simulink model "soc_swhw_fpga"  (R2021a)
settings: Solver=VariableStepAuto  StartTime=0.0  StopTime=stopTime  RelTol=1e-3  EnableMultiTasking=on
PreLoadFcn:
  | hsb.blkcb2.defineTypes;
undefined symbols (not defined in the file): a, b, Bias1, Bias2, c, frameSize, jsin, LUT_Z0, LUT_Z1, NumBits1, NumBits2, quantizationBits, sampleTime, SF, Slope1, Slope2
libraries: simulink x42, hdlsllib x24, embreciprocals x4, hwlogicconnlib x4, dsphdlxfrm x2, dsphdlmathfun x1
(part 2 of 2)

== system soc_swhw_fpga/FPGA Algorithm Wrapper/Output Adapter/Zero Chop ==
  validIn : Inport
  dataIn : Inport  Port=2
  AND : Logic  AllPortsSameDT=off  OutDataTypeStr=boolean
  Compare To Constant : simulink/Logic and Bit Operations/Compare To Constant  relop=<=  const=frameSize  OutDataTypeStr=boolean
  Compare To Constant1 : simulink/Logic and Bit Operations/Compare To Constant  relop=~=  const=0  OutDataTypeStr=boolean
  Enabled Counter1 : Subsystem  TreatAsAtomicUnit=on  mask(Counter){maxCount=(2 ^ (floor(log2(frameSize)) + 1)), sampleTime=-1}
      mask prompts: maxCount "Maximum count:"; sampleTime "Sample Time:"
  validOut : Outport
  dataOut : Outport  Port=2
  wires:
  AND/1 -> validOut/1
  Compare To Constant1/1 -> AND/2
  Enabled Counter1/1(count) -> Compare To Constant/1, Compare To Constant1/1
  Compare To Constant/1 -> AND/1
  validIn/1 -> Enabled Counter1/1(en)
  dataIn/1 -> dataOut/1

== system soc_swhw_fpga/FPGA Algorithm Wrapper/Feature Extraction/VAD/Enabled Counter ==
  en : Inport
  Compare To Constant : simulink/Logic and Bit Operations/Compare To Constant  relop===  const=maxCount  OutDataTypeStr=boolean
  Constant1 : Constant  Value=0  OutDataTypeStr=uint(floor(log2(maxCount))+1)  SampleTime=-1
  Delay One Step : Delay  DelayLength=1  InitialCondition=0
  Delay One Step1 : Delay  DelayLength=1  InitialCondition=0
  Increment Real World : simulink/Additional Math & Discrete/Additional Math: Increment - Decrement/Increment Real World
      settings: SourceProductBaseCode=SL
  Multiport Switch : MultiPortSwitch  DataPortOrder=Zero-based contiguous  Inputs=2  zeroidx=on
  Multiport Switch1 : MultiPortSwitch  DataPortOrder=Zero-based contiguous  Inputs=2  zeroidx=on
  Multiport Switch2 : MultiPortSwitch  DataPortOrder=Zero-based contiguous  Inputs=2  zeroidx=on
  count : Outport
  wires:
  en/1 -> Multiport Switch1/1, Multiport Switch/1
  Increment Real World/1 -> Multiport Switch/3
  Multiport Switch/1 -> Multiport Switch2/2, Multiport Switch1/3, Compare To Constant/1
  Delay One Step/1 -> Multiport Switch/2, Increment Real World/1
  Compare To Constant/1 -> Multiport Switch2/1
  Delay One Step1/1 -> Multiport Switch1/2
  Multiport Switch1/1 -> count/1, Delay One Step1/1
  Multiport Switch2/1 -> Delay One Step/1
  Constant1/1 -> Multiport Switch2/3

== system soc_swhw_fpga/FPGA Algorithm Wrapper/Feature Extraction/VAD/Pos Edge Detector ==
  q : Inport
  AND : Logic  AllPortsSameDT=off  OutDataTypeStr=boolean
  Delay1 : Delay  DelayLength=1
  XOR : Logic  Operator=XOR  AllPortsSameDT=off  OutDataTypeStr=boolean
  detected : Outport
  wires:
  XOR/1 -> AND/1
  Delay1/1 -> XOR/2
  q/1 -> XOR/1, AND/2, Delay1/1
  AND/1 -> detected/1

== system soc_swhw_fpga/FPGA Algorithm Wrapper/Feature Extraction/VAD/Pos Edge Detector1 ==
  q : Inport
  AND : Logic  AllPortsSameDT=off  OutDataTypeStr=boolean
  Delay1 : Delay  DelayLength=1
  XOR : Logic  Operator=XOR  AllPortsSameDT=off  OutDataTypeStr=boolean
  detected : Outport
  wires:
  XOR/1 -> AND/1
  Delay1/1 -> XOR/2
  q/1 -> XOR/1, AND/2, Delay1/1
  AND/1 -> detected/1

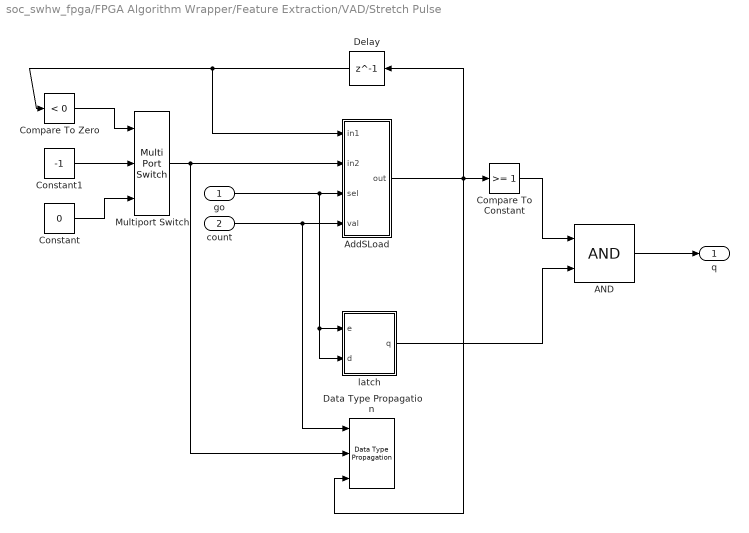
== system soc_swhw_fpga/FPGA Algorithm Wrapper/Feature Extraction/VAD/Stretch Pulse ==
  go : Inport  OutDataTypeStr=boolean
  count : Inport  Port=2
  AND : Logic  AllPortsSameDT=off  OutDataTypeStr=boolean
  AddSLoad : Subsystem
  Compare To Constant : simulink/Logic and Bit Operations/Compare To Constant  relop=>=  const=1  OutDataTypeStr=boolean
  Compare To Zero : simulink/Logic and Bit Operations/Compare To Zero  relop=<  OutDataTypeStr=boolean
  Constant : Constant  Value=0  OutDataTypeStr=fixdt(0,1,0)  SampleTime=-1
  Constant1 : Constant  Value=-1  OutDataTypeStr=fixdt(1,2,0)  SampleTime=-1
  Data Type Propagation : simulink/Signal Attributes/Data Type Propagation  PropDataType=fixdt(1, 16)  IfRefDouble=double  IfRefSingle=single  IsSigned=IsSigned1 or IsSigned2  NumBitsBase=max([NumBits1 NumBits2])  NumBitsMult=1  NumBitsAdd=1  NumBitsAllowFinal=1:128  PropScaling=2^-10  ValuesUsedBestPrec=[5 -7]  SlopeBase=max([Slope1 Slope2])  SlopeMult=1  SlopeAdd=0  BiasBase=Bias1+Bias2  BiasMult=1  BiasAdd=0
      settings: SourceProductBaseCode=SL
  Delay : Delay  DelayLength=1
  Multiport Switch : MultiPortSwitch  DataPortOrder=Zero-based contiguous  Inputs=2  zeroidx=on
  latch : Subsystem
  q : Outport
  wires:
  AddSLoad/1(out) -> Data Type Propagation/3, Compare To Constant/1, Delay/1
  Constant/1 -> Multiport Switch/3
  Delay/1 -> Compare To Zero/1, AddSLoad/1(in1)
  latch/1(q) -> AND/2
  Constant1/1 -> Multiport Switch/2
  Multiport Switch/1 -> Data Type Propagation/2, AddSLoad/2(in2)
  Compare To Zero/1 -> Multiport Switch/1
  Compare To Constant/1 -> AND/1
  go/1 -> latch/1(e), latch/2(d), AddSLoad/3(sel)
  AND/1 -> q/1
  count/1 -> Data Type Propagation/1, AddSLoad/4(val)

== system soc_swhw_fpga/FPGA Algorithm Wrapper/Feature Extraction/VAD/bitFuse ==
  q : Inport
  Delay : Delay  DelayLength=1
  Multiport Switch : MultiPortSwitch  DataPortOrder=Zero-based contiguous  Inputs=2  zeroidx=on
  tripped : Outport
  wires:
  Delay/1 -> Multiport Switch/3, Multiport Switch/1
  Multiport Switch/1 -> tripped/1, Delay/1
  q/1 -> Multiport Switch/2

== system soc_swhw_fpga/FPGA Algorithm Wrapper/Feature Extraction/aPosterioriSNR/Frame Fuse ==
  validIn : Inport
  1bit Counter : hdlsllib/Sources/HDL Counter  CountType=Count limited  CountInit=0  CountStep=1  CountMax=1  CountFromType=Initial value  CountFrom=0  CountResetPort=off  CountLoadPort=off  CountEnbPort=on  CountDirPort=off  CountHitOutputPort=off  CountDataType=Unsigned  CountWordLen=1  CountFracLen=0  CountSampTime=1
  Constant : Constant  Value=0  OutDataTypeStr=fixdt(0, 1, 0)  SampleTime=sampleTime
  Delay : Delay  DelayLength=1
  Multiport Switch : MultiPortSwitch  DataPortOrder=Zero-based contiguous  Inputs=2  zeroidx=on
  Pulse Divider : Subsystem  mask{N=ceil(log2(frameSize)) - 1}
  tripped : Outport
  wires:
  1bit Counter/1 -> Delay/1
  Constant/1 -> Multiport Switch/3
  Delay/1 -> Multiport Switch/1, tripped/1
  Pulse Divider/1(q) -> Multiport Switch/2
  validIn/1 -> Pulse Divider/1(In1)
  Multiport Switch/1 -> 1bit Counter/1

== system soc_swhw_fpga/FPGA Algorithm Wrapper/Feature Extraction/aPosterioriSNR/Zero Eliminator ==
  in : Inport
  Compare To Zero : simulink/Logic and Bit Operations/Compare To Zero  relop===  OutDataTypeStr=boolean
  Constant : Constant  OutDataTypeStr=fixdt(0, 1, 0)
  Multiport Switch6 : MultiPortSwitch  DataPortOrder=Zero-based contiguous  Inputs=2  zeroidx=on
  out : Outport
  wires:
  Multiport Switch6/1 -> out/1
  Compare To Zero/1 -> Multiport Switch6/1
  Constant/1 -> Multiport Switch6/3
  in/1 -> Multiport Switch6/2, Compare To Zero/1

== system soc_swhw_fpga/FPGA Algorithm Wrapper/Feature Extraction/aPosterioriSNR/Zero Eliminator1 ==
  in : Inport
  Compare To Zero : simulink/Logic and Bit Operations/Compare To Zero  relop===  OutDataTypeStr=boolean
  Constant : Constant  OutDataTypeStr=fixdt(0, 1, 0)
  Multiport Switch6 : MultiPortSwitch  DataPortOrder=Zero-based contiguous  Inputs=2  zeroidx=on
  out : Outport
  wires:
  in/1 -> Compare To Zero/1, Multiport Switch6/2
  Constant/1 -> Multiport Switch6/3
  Compare To Zero/1 -> Multiport Switch6/1
  Multiport Switch6/1 -> out/1

== system soc_swhw_fpga/FPGA Algorithm Wrapper/Feature Extraction/aPrioriSNR/Frame Fuse ==
  validIn : Inport
  1bit Counter : hdlsllib/Sources/HDL Counter  CountType=Count limited  CountInit=0  CountStep=1  CountMax=1  CountFromType=Initial value  CountFrom=0  CountResetPort=off  CountLoadPort=off  CountEnbPort=on  CountDirPort=off  CountHitOutputPort=off  CountDataType=Unsigned  CountWordLen=1  CountFracLen=0  CountSampTime=1
  Constant : Constant  Value=0  OutDataTypeStr=fixdt(0, 1, 0)  SampleTime=sampleTime
  Delay : Delay  DelayLength=1
  Multiport Switch : MultiPortSwitch  DataPortOrder=Zero-based contiguous  Inputs=2  zeroidx=on
  Pulse Divider : Subsystem  mask{N=ceil(log2(frameSize)) - 1}
  tripped : Outport
  wires:
  1bit Counter/1 -> Delay/1
  Constant/1 -> Multiport Switch/3
  Delay/1 -> Multiport Switch/1, tripped/1
  Pulse Divider/1(q) -> Multiport Switch/2
  validIn/1 -> Pulse Divider/1(In1)
  Multiport Switch/1 -> 1bit Counter/1

== system soc_swhw_fpga/FPGA Algorithm Wrapper/Input Adapter/Hamming Window/Enabled Counter ==
  en : Inport
  Compare To Constant : simulink/Logic and Bit Operations/Compare To Constant  relop===  const=maxCount  OutDataTypeStr=boolean
  Constant1 : Constant  Value=0  OutDataTypeStr=uint(floor(log2(maxCount))+1)  SampleTime=-1
  Delay One Step : Delay  DelayLength=1  InitialCondition=0
  Delay One Step1 : Delay  DelayLength=1  InitialCondition=0
  Increment Real World : simulink/Additional Math & Discrete/Additional Math: Increment - Decrement/Increment Real World
      settings: SourceProductBaseCode=SL
  Multiport Switch : MultiPortSwitch  DataPortOrder=Zero-based contiguous  Inputs=2  zeroidx=on
  Multiport Switch1 : MultiPortSwitch  DataPortOrder=Zero-based contiguous  Inputs=2  zeroidx=on
  Multiport Switch2 : MultiPortSwitch  DataPortOrder=Zero-based contiguous  Inputs=2  zeroidx=on
  count : Outport
  wires:
  en/1 -> Multiport Switch1/1, Multiport Switch/1
  Increment Real World/1 -> Multiport Switch/3
  Multiport Switch/1 -> Multiport Switch2/2, Multiport Switch1/3, Compare To Constant/1
  Delay One Step/1 -> Increment Real World/1, Multiport Switch/2
  Compare To Constant/1 -> Multiport Switch2/1
  Delay One Step1/1 -> Multiport Switch1/2
  Multiport Switch1/1 -> count/1, Delay One Step1/1
  Multiport Switch2/1 -> Delay One Step/1
  Constant1/1 -> Multiport Switch2/3

== system soc_swhw_fpga/FPGA Algorithm Wrapper/Input Adapter/Single-Sided Spectrum/Enabled Counter ==
  en : Inport
  Compare To Constant : simulink/Logic and Bit Operations/Compare To Constant  relop===  const=maxCount  OutDataTypeStr=boolean
  Constant1 : Constant  Value=0  OutDataTypeStr=uint(floor(log2(maxCount))+1)  SampleTime=-1
  Delay One Step : Delay  DelayLength=1  InitialCondition=0
  Delay One Step1 : Delay  DelayLength=1  InitialCondition=0
  Increment Real World : simulink/Additional Math & Discrete/Additional Math: Increment - Decrement/Increment Real World
      settings: SourceProductBaseCode=SL
  Multiport Switch : MultiPortSwitch  DataPortOrder=Zero-based contiguous  Inputs=2  zeroidx=on
  Multiport Switch1 : MultiPortSwitch  DataPortOrder=Zero-based contiguous  Inputs=2  zeroidx=on
  Multiport Switch2 : MultiPortSwitch  DataPortOrder=Zero-based contiguous  Inputs=2  zeroidx=on
  count : Outport
  wires:
  en/1 -> Multiport Switch1/1, Multiport Switch/1
  Increment Real World/1 -> Multiport Switch/3
  Multiport Switch/1 -> Multiport Switch2/2, Multiport Switch1/3, Compare To Constant/1
  Delay One Step/1 -> Multiport Switch/2, Increment Real World/1
  Compare To Constant/1 -> Multiport Switch2/1
  Delay One Step1/1 -> Multiport Switch1/2
  Multiport Switch1/1 -> count/1, Delay One Step1/1
  Multiport Switch2/1 -> Delay One Step/1
  Constant1/1 -> Multiport Switch2/3

== system soc_swhw_fpga/FPGA Algorithm Wrapper/Input Adapter/Zero Pad/Enabled Counter ==
  en : Inport
  Compare To Constant : simulink/Logic and Bit Operations/Compare To Constant  relop===  const=maxCount  OutDataTypeStr=boolean
  Constant1 : Constant  Value=0  OutDataTypeStr=uint(floor(log2(maxCount))+1)  SampleTime=-1
  Delay One Step : Delay  DelayLength=1  InitialCondition=0
  Delay One Step1 : Delay  DelayLength=1  InitialCondition=0
  Increment Real World : simulink/Additional Math & Discrete/Additional Math: Increment - Decrement/Increment Real World
      settings: SourceProductBaseCode=SL
  Multiport Switch : MultiPortSwitch  DataPortOrder=Zero-based contiguous  Inputs=2  zeroidx=on
  Multiport Switch1 : MultiPortSwitch  DataPortOrder=Zero-based contiguous  Inputs=2  zeroidx=on
  Multiport Switch2 : MultiPortSwitch  DataPortOrder=Zero-based contiguous  Inputs=2  zeroidx=on
  count : Outport
  wires:
  en/1 -> Multiport Switch1/1, Multiport Switch/1
  Increment Real World/1 -> Multiport Switch/3
  Multiport Switch/1 -> Multiport Switch2/2, Multiport Switch1/3, Compare To Constant/1
  Delay One Step/1 -> Increment Real World/1, Multiport Switch/2
  Compare To Constant/1 -> Multiport Switch2/1
  Delay One Step1/1 -> Multiport Switch1/2
  Multiport Switch1/1 -> count/1, Delay One Step1/1
  Multiport Switch2/1 -> Delay One Step/1
  Constant1/1 -> Multiport Switch2/3

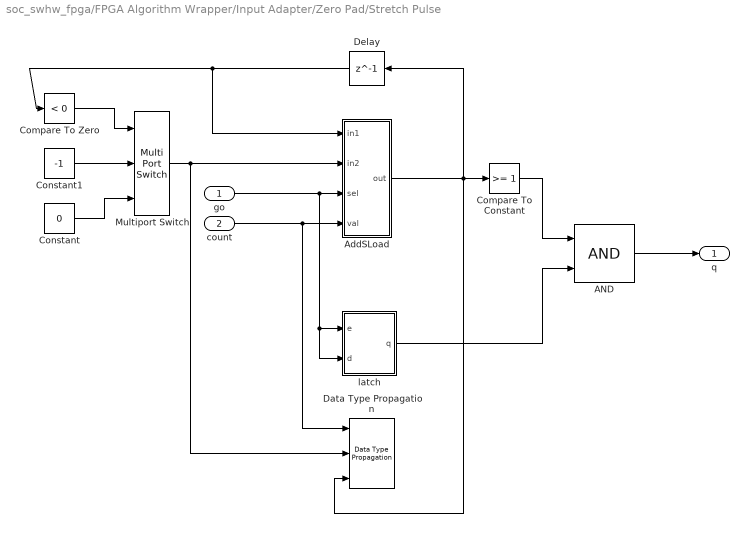
== system soc_swhw_fpga/FPGA Algorithm Wrapper/Input Adapter/Zero Pad/Stretch Pulse ==
  go : Inport  OutDataTypeStr=boolean
  count : Inport  Port=2
  AND : Logic  AllPortsSameDT=off  OutDataTypeStr=boolean
  AddSLoad : Subsystem
  Compare To Constant : simulink/Logic and Bit Operations/Compare To Constant  relop=>=  const=1  OutDataTypeStr=boolean
  Compare To Zero : simulink/Logic and Bit Operations/Compare To Zero  relop=<  OutDataTypeStr=boolean
  Constant : Constant  Value=0  OutDataTypeStr=fixdt(0,1,0)  SampleTime=-1
  Constant1 : Constant  Value=-1  OutDataTypeStr=fixdt(1,2,0)  SampleTime=-1
  Data Type Propagation : simulink/Signal Attributes/Data Type Propagation  PropDataType=fixdt(1, 16)  IfRefDouble=double  IfRefSingle=single  IsSigned=IsSigned1 or IsSigned2  NumBitsBase=max([NumBits1 NumBits2])  NumBitsMult=1  NumBitsAdd=1  NumBitsAllowFinal=1:128  PropScaling=2^-10  ValuesUsedBestPrec=[5 -7]  SlopeBase=max([Slope1 Slope2])  SlopeMult=1  SlopeAdd=0  BiasBase=Bias1+Bias2  BiasMult=1  BiasAdd=0
      settings: SourceProductBaseCode=SL
  Delay : Delay  DelayLength=1
  Multiport Switch : MultiPortSwitch  DataPortOrder=Zero-based contiguous  Inputs=2  zeroidx=on
  latch : Subsystem
  q : Outport
  wires:
  AddSLoad/1(out) -> Data Type Propagation/3, Compare To Constant/1, Delay/1
  Constant/1 -> Multiport Switch/3
  Delay/1 -> Compare To Zero/1, AddSLoad/1(in1)
  latch/1(q) -> AND/2
  Constant1/1 -> Multiport Switch/2
  Multiport Switch/1 -> Data Type Propagation/2, AddSLoad/2(in2)
  Compare To Zero/1 -> Multiport Switch/1
  Compare To Constant/1 -> AND/1
  go/1 -> latch/1(e), latch/2(d), AddSLoad/3(sel)
  AND/1 -> q/1
  count/1 -> Data Type Propagation/1, AddSLoad/4(val)

== system soc_swhw_fpga/FPGA Algorithm Wrapper/Input Adapter/Zero Pad/pos Edge Detector1 ==
  q : Inport
  AND : Logic  AllPortsSameDT=off  OutDataTypeStr=boolean
  Delay1 : Delay  DelayLength=1
  XOR : Logic  Operator=XOR  AllPortsSameDT=off  OutDataTypeStr=boolean
  detected : Outport
  wires:
  XOR/1 -> AND/1
  Delay1/1 -> XOR/2
  q/1 -> XOR/1, AND/2, Delay1/1
  AND/1 -> detected/1

== system soc_swhw_fpga/FPGA Algorithm Wrapper/Output Adapter/Spectrum Mirror/Pulse Multiplier ==
  go : Inport
  AddSLoad : Subsystem
  Cast To Boolean : DataTypeConversion  OutDataTypeStr=boolean  RndMeth=Simplest
  Constant5 : Constant  Value=2^N  OutDataTypeStr=ufix(N + 1)  SampleTime=sampleTime
  Data Type Conversion : DataTypeConversion  OutDataTypeStr=fixdt(0, 1, 0)  RndMeth=Simplest
  Delay : Delay  DelayLength=1
  Delay1 : Delay  DelayLength=1
  Extract Bits : simulink/Logic and Bit Operations/Extract Bits  bitsToExtract=Range of bits  numBits=1  bitIdxRange=[N N]  outScalingMode=Treat bit field as an integer
  q : Outport
  wires:
  go/1 -> AddSLoad/3(sel)
  AddSLoad/1(out) -> Delay1/1, Extract Bits/1
  Delay1/1 -> AddSLoad/1(in1)
  Extract Bits/1 -> Cast To Boolean/1, Delay/1
  Data Type Conversion/1 -> AddSLoad/2(in2)
  Delay/1 -> Data Type Conversion/1
  Constant5/1 -> AddSLoad/4(val)
  Cast To Boolean/1 -> q/1

== system soc_swhw_fpga/FPGA Algorithm Wrapper/Output Adapter/Spectrum Mirror/addressCounter0 ==
  en : Inport
  Constant4 : Constant  OutDataTypeStr=fixdt(0, 1, 0)  SampleTime=sampleTime
  Enabled Counter : Subsystem  TreatAsAtomicUnit=on  mask(Counter){maxCount=2 ^ floor(log2(frameSize)), sampleTime=-1}
      mask prompts: maxCount "Maximum count:"; sampleTime "Sample Time:"
  Subtract3 : Sum  Inputs=+-  RndMeth=Simplest  OutDataTypeStr=Inherit: Same as first input
  addr : Outport
  wires:
  Subtract3/1 -> addr/1
  Constant4/1 -> Subtract3/2
  Enabled Counter/1(count) -> Subtract3/1
  en/1 -> Enabled Counter/1(en)

== system soc_swhw_fpga/FPGA Algorithm Wrapper/Output Adapter/Spectrum Mirror/addressCounter1 ==
  en : Inport
  Constant4 : Constant  OutDataTypeStr=fixdt(0, 1, 0)  SampleTime=sampleTime
  Enabled Counter : Subsystem  TreatAsAtomicUnit=on  mask(Counter){maxCount=2 ^ (floor(log2(frameSize)) + 1), sampleTime=-1}
      mask prompts: maxCount "Maximum count:"; sampleTime "Sample Time:"
  Subtract3 : Sum  Inputs=+-  OutDataTypeStr=fixdt(0,(floor(log2(frameSize)) + 1),0)  RndMeth=Simplest
  addr : Outport
  wires:
  Subtract3/1 -> addr/1
  Constant4/1 -> Subtract3/2
  Enabled Counter/1(count) -> Subtract3/1
  en/1 -> Enabled Counter/1(en)

== system soc_swhw_fpga/FPGA Algorithm Wrapper/Output Adapter/Spectrum Mirror/pos Edge Detector1 ==
  q : Inport
  AND : Logic  AllPortsSameDT=off  OutDataTypeStr=boolean
  Delay1 : Delay  DelayLength=1
  XOR : Logic  Operator=XOR  AllPortsSameDT=off  OutDataTypeStr=boolean
  detected : Outport
  wires:
  XOR/1 -> AND/1
  Delay1/1 -> XOR/2
  q/1 -> XOR/1, AND/2, Delay1/1
  AND/1 -> detected/1

== system soc_swhw_fpga/FPGA Algorithm Wrapper/Output Adapter/Zero Chop/Enabled Counter1 ==
  en : Inport
  Compare To Constant : simulink/Logic and Bit Operations/Compare To Constant  relop===  const=maxCount  OutDataTypeStr=boolean
  Constant1 : Constant  Value=0  OutDataTypeStr=uint(floor(log2(maxCount))+1)  SampleTime=-1
  Delay One Step : Delay  DelayLength=1  InitialCondition=0
  Delay One Step1 : Delay  DelayLength=1  InitialCondition=0
  Increment Real World : simulink/Additional Math & Discrete/Additional Math: Increment - Decrement/Increment Real World
      settings: SourceProductBaseCode=SL
  Multiport Switch : MultiPortSwitch  DataPortOrder=Zero-based contiguous  Inputs=2  zeroidx=on
  Multiport Switch1 : MultiPortSwitch  DataPortOrder=Zero-based contiguous  Inputs=2  zeroidx=on
  Multiport Switch2 : MultiPortSwitch  DataPortOrder=Zero-based contiguous  Inputs=2  zeroidx=on
  count : Outport
  wires:
  en/1 -> Multiport Switch1/1, Multiport Switch/1
  Increment Real World/1 -> Multiport Switch/3
  Multiport Switch/1 -> Multiport Switch2/2, Multiport Switch1/3, Compare To Constant/1
  Delay One Step/1 -> Increment Real World/1, Multiport Switch/2
  Compare To Constant/1 -> Multiport Switch2/1
  Delay One Step1/1 -> Multiport Switch1/2
  Multiport Switch1/1 -> count/1, Delay One Step1/1
  Multiport Switch2/1 -> Delay One Step/1
  Constant1/1 -> Multiport Switch2/3

== system soc_swhw_fpga/FPGA Algorithm Wrapper/Feature Extraction/VAD/Stretch Pulse/AddSLoad ==
  in1 : Inport
  in2 : Inport  Port=2
  sel : Inport  Port=3
  val : Inport  Port=4
  Add1 : Sum  RndMeth=Simplest
  Multiport Switch : MultiPortSwitch  DataPortOrder=Zero-based contiguous  Inputs=2  zeroidx=on
  out : Outport
  wires:
  Multiport Switch/1 -> out/1
  Add1/1 -> Multiport Switch/2
  val/1 -> Multiport Switch/3
  sel/1 -> Multiport Switch/1
  in2/1 -> Add1/2
  in1/1 -> Add1/1

== system soc_swhw_fpga/FPGA Algorithm Wrapper/Feature Extraction/VAD/Stretch Pulse/latch ==
  e : Inport
  d : Inport  Port=2
  Delay : Delay  DelayLength=1
  Multiport Switch : MultiPortSwitch  DataPortOrder=Zero-based contiguous  Inputs=2  zeroidx=on
  q : Outport
  wires:
  Delay/1 -> Multiport Switch/2
  e/1 -> Multiport Switch/1
  d/1 -> Multiport Switch/3
  Multiport Switch/1 -> Delay/1, q/1

== system soc_swhw_fpga/FPGA Algorithm Wrapper/Feature Extraction/aPosterioriSNR/Frame Fuse/Pulse Divider ==
  In1 : Inport
  Bit Slice : hdlsllib/Logic and Bit Operations/Bit Slice  lidx=N  ridx=N
      settings: SourceProductBaseCode=SL
  Edge Detector : Subsystem
  HDL Counter : hdlsllib/Sources/HDL Counter  CountType=Count limited  CountInit=0  CountStep=1  CountMax=2 ^ (N + 1) - 1  CountFromType=Initial value  CountFrom=0  CountResetPort=off  CountLoadPort=off  CountEnbPort=on  CountDirPort=off  CountHitOutputPort=off  CountDataType=Unsigned  CountWordLen=N + 1  CountFracLen=0  CountSampTime=1
  q : Outport
  wires:
  HDL Counter/1 -> Bit Slice/1
  In1/1 -> HDL Counter/1
  Bit Slice/1 -> Edge Detector/1(d)
  Edge Detector/1(q) -> q/1

== system soc_swhw_fpga/FPGA Algorithm Wrapper/Feature Extraction/aPrioriSNR/Frame Fuse/Pulse Divider ==
  In1 : Inport
  Bit Slice : hdlsllib/Logic and Bit Operations/Bit Slice  lidx=N  ridx=N
      settings: SourceProductBaseCode=SL
  Edge Detector : Subsystem
  HDL Counter : hdlsllib/Sources/HDL Counter  CountType=Count limited  CountInit=0  CountStep=1  CountMax=2 ^ (N + 1) - 1  CountFromType=Initial value  CountFrom=0  CountResetPort=off  CountLoadPort=off  CountEnbPort=on  CountDirPort=off  CountHitOutputPort=off  CountDataType=Unsigned  CountWordLen=N + 1  CountFracLen=0  CountSampTime=1
  q : Outport
  wires:
  HDL Counter/1 -> Bit Slice/1
  In1/1 -> HDL Counter/1
  Bit Slice/1 -> Edge Detector/1(d)
  Edge Detector/1(q) -> q/1

== system soc_swhw_fpga/FPGA Algorithm Wrapper/Input Adapter/Zero Pad/Stretch Pulse/AddSLoad ==
  in1 : Inport
  in2 : Inport  Port=2
  sel : Inport  Port=3
  val : Inport  Port=4
  Add1 : Sum  RndMeth=Simplest
  Multiport Switch : MultiPortSwitch  DataPortOrder=Zero-based contiguous  Inputs=2  zeroidx=on
  out : Outport
  wires:
  Multiport Switch/1 -> out/1
  Add1/1 -> Multiport Switch/2
  val/1 -> Multiport Switch/3
  sel/1 -> Multiport Switch/1
  in2/1 -> Add1/2
  in1/1 -> Add1/1

== system soc_swhw_fpga/FPGA Algorithm Wrapper/Input Adapter/Zero Pad/Stretch Pulse/latch ==
  e : Inport
  d : Inport  Port=2
  Delay : Delay  DelayLength=1
  Multiport Switch : MultiPortSwitch  DataPortOrder=Zero-based contiguous  Inputs=2  zeroidx=on
  q : Outport
  wires:
  Delay/1 -> Multiport Switch/2
  e/1 -> Multiport Switch/1
  d/1 -> Multiport Switch/3
  Multiport Switch/1 -> Delay/1, q/1

== system soc_swhw_fpga/FPGA Algorithm Wrapper/Output Adapter/Spectrum Mirror/Pulse Multiplier/AddSLoad ==
  in1 : Inport
  in2 : Inport  Port=2
  sel : Inport  Port=3
  val : Inport  Port=4
  Add1 : Sum  RndMeth=Simplest
  Multiport Switch : MultiPortSwitch  DataPortOrder=Zero-based contiguous  Inputs=2  zeroidx=on  RndMeth=Simplest
  out : Outport
  wires:
  Multiport Switch/1 -> out/1
  Add1/1 -> Multiport Switch/2
  val/1 -> Multiport Switch/3
  sel/1 -> Multiport Switch/1
  in2/1 -> Add1/2
  in1/1 -> Add1/1

== system soc_swhw_fpga/FPGA Algorithm Wrapper/Output Adapter/Spectrum Mirror/addressCounter0/Enabled Counter ==
  en : Inport
  Compare To Constant : simulink/Logic and Bit Operations/Compare To Constant  relop===  const=maxCount  OutDataTypeStr=boolean
  Constant1 : Constant  Value=0  OutDataTypeStr=uint(floor(log2(maxCount))+1)  SampleTime=-1
  Delay One Step : Delay  DelayLength=1  InitialCondition=0
  Delay One Step1 : Delay  DelayLength=1  InitialCondition=0
  Increment Real World : simulink/Additional Math & Discrete/Additional Math: Increment - Decrement/Increment Real World
      settings: SourceProductBaseCode=SL
  Multiport Switch : MultiPortSwitch  DataPortOrder=Zero-based contiguous  Inputs=2  zeroidx=on
  Multiport Switch1 : MultiPortSwitch  DataPortOrder=Zero-based contiguous  Inputs=2  zeroidx=on
  Multiport Switch2 : MultiPortSwitch  DataPortOrder=Zero-based contiguous  Inputs=2  zeroidx=on
  count : Outport
  wires:
  en/1 -> Multiport Switch1/1, Multiport Switch/1
  Increment Real World/1 -> Multiport Switch/3
  Multiport Switch/1 -> Multiport Switch2/2, Multiport Switch1/3, Compare To Constant/1
  Delay One Step/1 -> Increment Real World/1, Multiport Switch/2
  Compare To Constant/1 -> Multiport Switch2/1
  Delay One Step1/1 -> Multiport Switch1/2
  Multiport Switch1/1 -> count/1, Delay One Step1/1
  Multiport Switch2/1 -> Delay One Step/1
  Constant1/1 -> Multiport Switch2/3

== system soc_swhw_fpga/FPGA Algorithm Wrapper/Output Adapter/Spectrum Mirror/addressCounter1/Enabled Counter ==
  en : Inport
  Compare To Constant : simulink/Logic and Bit Operations/Compare To Constant  relop===  const=maxCount  OutDataTypeStr=boolean
  Constant1 : Constant  Value=0  OutDataTypeStr=uint(floor(log2(maxCount))+1)  SampleTime=-1
  Delay One Step : Delay  DelayLength=1  InitialCondition=0
  Delay One Step1 : Delay  DelayLength=1  InitialCondition=0
  Increment Real World : simulink/Additional Math & Discrete/Additional Math: Increment - Decrement/Increment Real World
      settings: SourceProductBaseCode=SL
  Multiport Switch : MultiPortSwitch  DataPortOrder=Zero-based contiguous  Inputs=2  zeroidx=on
  Multiport Switch1 : MultiPortSwitch  DataPortOrder=Zero-based contiguous  Inputs=2  zeroidx=on
  Multiport Switch2 : MultiPortSwitch  DataPortOrder=Zero-based contiguous  Inputs=2  zeroidx=on
  count : Outport
  wires:
  en/1 -> Multiport Switch1/1, Multiport Switch/1
  Increment Real World/1 -> Multiport Switch/3
  Multiport Switch/1 -> Multiport Switch2/2, Multiport Switch1/3, Compare To Constant/1
  Delay One Step/1 -> Increment Real World/1, Multiport Switch/2
  Compare To Constant/1 -> Multiport Switch2/1
  Delay One Step1/1 -> Multiport Switch1/2
  Multiport Switch1/1 -> count/1, Delay One Step1/1
  Multiport Switch2/1 -> Delay One Step/1
  Constant1/1 -> Multiport Switch2/3

== system soc_swhw_fpga/FPGA Algorithm Wrapper/Feature Extraction/aPosterioriSNR/Frame Fuse/Pulse Divider/Edge Detector ==
  d : Inport
  Delay : Delay  DelayLength=1
  XOR : Logic  Operator=XOR  AllPortsSameDT=off  OutDataTypeStr=boolean
  q : Outport
  wires:
  Delay/1 -> XOR/2
  d/1 -> XOR/1, Delay/1
  XOR/1 -> q/1

== system soc_swhw_fpga/FPGA Algorithm Wrapper/Feature Extraction/aPrioriSNR/Frame Fuse/Pulse Divider/Edge Detector ==
  d : Inport
  Delay : Delay  DelayLength=1
  XOR : Logic  Operator=XOR  AllPortsSameDT=off  OutDataTypeStr=boolean
  q : Outport
  wires:
  Delay/1 -> XOR/2
  d/1 -> XOR/1, Delay/1
  XOR/1 -> q/1
